simulink model "save_sourcegen"  (R2017a)
settings: Solver=VariableStepAuto  StartTime=0.0  StopTime=10  RelTol=1e-3
libraries: simulink x2
settings Model: Creator=brunolnetto  LastModifiedBy=brunolnetto

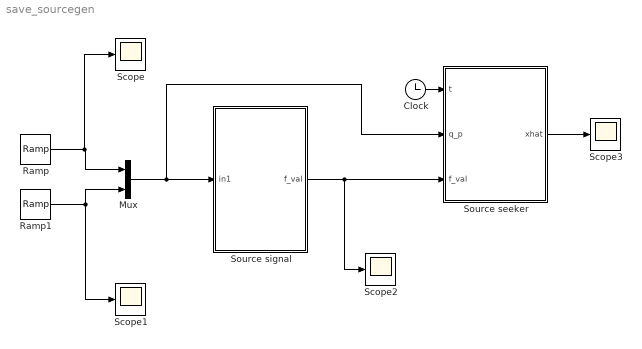
== system save_sourcegen ==
  Clock : Clock
  Mux : Mux  Inputs=2
  Ramp : simulink/Sources/Ramp  slope=-1  start=0  X0=1
  Ramp1 : simulink/Sources/Ramp  slope=-1  start=0  X0=1
  Scope{,1..3} (4 alike) : Scope
  Source seeker : Subsystem
  Source signal : MATLAB Function  TreatAsAtomicUnit=on
  wires:
  Clock/1 -> Source seeker/1(t)
  Source seeker/1(xhat) -> Scope3/1
  Mux/1 -> Source seeker/2(q_p), Source signal/1(in1)
  Ramp/1 -> Scope/1, Mux/1
  Ramp1/1 -> Scope1/1, Mux/2
  Source signal/1(f_val) -> Source seeker/3(f_val), Scope2/1

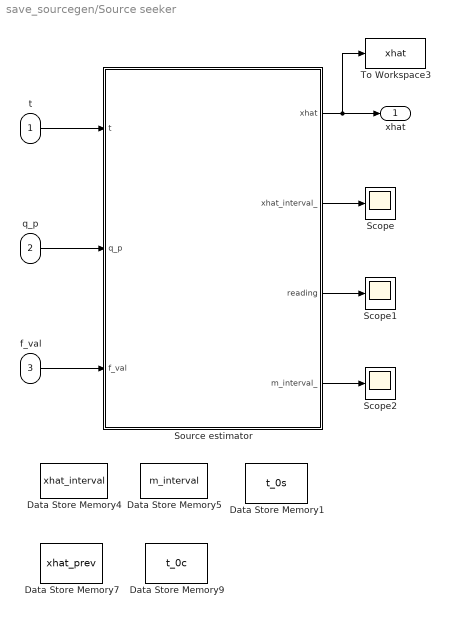
== system save_sourcegen/Source seeker ==
  t : Inport
  q_p : Inport  Port=2
  f_val : Inport  Port=3
  Data Store Memory1 : DataStoreMemory  DataStoreName=t_0s  ReadBeforeWriteMsg=warning  WriteAfterWriteMsg=warning  WriteAfterReadMsg=warning  ShowAdditionalParam=off  OutDataTypeStr=double
  Data Store Memory4 : DataStoreMemory  DataStoreName=xhat_interval  ReadBeforeWriteMsg=warning  WriteAfterWriteMsg=warning  WriteAfterReadMsg=warning  InitialValue=xhat0  ShowAdditionalParam=off  OutDataTypeStr=double  Dimensions=[2, 1]
  Data Store Memory5 : DataStoreMemory  DataStoreName=m_interval  ReadBeforeWriteMsg=warning  WriteAfterWriteMsg=warning  WriteAfterReadMsg=warning  ShowAdditionalParam=off  OutDataTypeStr=double
  Data Store Memory7 : DataStoreMemory  DataStoreName=xhat_prev  ReadBeforeWriteMsg=warning  WriteAfterWriteMsg=warning  WriteAfterReadMsg=warning  InitialValue=xhat0  ShowAdditionalParam=off  OutDataTypeStr=double
  Data Store Memory9 : DataStoreMemory  DataStoreName=t_0c  ReadBeforeWriteMsg=warning  WriteAfterWriteMsg=warning  WriteAfterReadMsg=warning  ShowAdditionalParam=off  OutDataTypeStr=double
  Scope : Scope
  Scope1 : Scope
  Scope2 : Scope
  Source estimator : MATLAB Function  TreatAsAtomicUnit=on
  To Workspace3 : ToWorkspace  VariableName=xhat  SaveFormat=Structure With Time  SampleTime=-1
  xhat : Outport
  wires:
  Source estimator/1(xhat) -> To Workspace3/1, xhat/1
  t/1 -> Source estimator/1(t)
  q_p/1 -> Source estimator/2(q_p)
  f_val/1 -> Source estimator/3(f_val)
  Source estimator/2(xhat_interval_) -> Scope/1
  Source estimator/3(reading) -> Scope1/1
  Source estimator/4(m_interval_) -> Scope2/1

== matlab function save_sourcegen/Source seeker/Source estimator ==
  data: t input; q_p input; xhat_interval data_store_memory; m_interval data_store_memory; xhat_prev data_store_memory; t_0c data_store_memory; f_val input; xhat output; xhat_interval_ output; reading output; m_interval_ output; source_params parameter; t_0s data_store_memory
function [xhat, xhat_interval_, reading, m_interval_] = ...
            source_estimation(t, q_p, f_val, source_params)
    
    global t_0c t_0s xhat_prev m_interval xhat_interval;
    
    % Source seeking parameters
    nu = source_params.nu;
    lambda = source_params.lambda;
    T_cur = source_params.T_cur;
    T_sample = source_params.T_sample;
    devval = source_params.devval;
    
    % Current position
    x_curr = q_p(1:2, 1);
    
    n = length(x_curr);
    
    % Update source estimation window
    if(t - t_0c > T_cur)
        t_0c = t;
        
        z = gaussianrnd([0; 0], devval);
        xhat_prev = xhat_interval + z;
    
    elseif(t - t_0s > T_sample)
        t_0s = t;
        
        % Barycenter along the trajectory
        e_i = exp(-nu*f_val);
        
        bary_num = lambda*m_interval*xhat_interval + x_curr*e_i;
        bary_den = lambda*m_interval + e_i;
        
        xhat_interval = bary_num/bary_den;
        m_interval = bary_den;
    
    end
    
    xhat = xhat_prev;
    xhat_interval_ = xhat_interval;
    m_interval_ = m_interval;
    reading = f_val;
end

== matlab function save_sourcegen/Source signal ==
  data: in1 input; f_val output
function f_val = source_signal(in1)

%    This function was generated by the Symbolic Math Toolbox version 7.2.

%    16-Feb-2021 18:42:54



x = in1(1,:);

y = in1(2,:);

f_val = x.^2+y.^2;

end
